simulink model "S32K39_FaultLogic_NXP_Codegen"  (R2024a)
settings: Solver=FixedStepAuto  StartTime=0.0  StopTime=10.0  FixedStep=1  RelTol=1e-3
PreLoadFcn:
  | % NXP_MBDT_S32K3 callback: DO NOT REMOVE
  | mbd_s32k3.common.nxp.model_callbacks.preLoadFcn();
PostLoadFcn:
  | % NXP_MBDT_S32K3 callback: DO NOT REMOVE
  | mbd_s32k3.common.nxp.model_callbacks.postLoadFcn();
InitFcn:
  | % NXP_MBDT_S32K3 callback: DO NOT REMOVE
  | mbd_s32k3.common.nxp.model_callbacks.initFcn();
settings Model: DataDictionary=S32K39_FaultLogic_NXP_Codegen.sldd  Creator=nxf64875  LastModifiedBy=nxf64875
settings DataIOCC: SaveOutput=off  SaveTime=off
settings OptimizationCC: EnhancedBackFolding=on  PassReuseOutputArgsAs=Individual arguments  ZeroExternalMemoryAtStartup=off  ZeroInternalMemoryAtStartup=off  MaxStackSize=64  OptimizeBlockOrder=speed  DifferentSizesBufferReuse=on  OptimizationCustomize=off  EfficientTunableParamExpr=on
settings DebuggingCC: ParameterTunabilityLossMsg=error
settings HardwareCC: ProdBitPerPointer=32  ProdBitPerSizeT=32  ProdBitPerPtrDiffT=32  ProdLargestAtomicInteger=Long  ProdLargestAtomicFloat=Double  ProdWordSize=32  ProdHWDeviceType=ARM Compatible->ARM Cortex
settings SFSimCC: MATLABDynamicMemAlloc=off
settings RTWCC: Description=Embedded Coder  SystemTargetFile=ert.tlc  HardwareBoard=NXP S32K3xx  TemplateMakefile=ert_default_tmf  Toolchain=S32DS GCC  BuildConfiguration=Faster Runs  CodeExecutionProfiling=on  CodeProfilingInstrumentation=coarse
settings CodeAppCC: ForceParamTrailComments=on  IgnoreCustomStorageClasses=off  OperatorAnnotations=on  SimulinkDataObjDesc=on  SFDataObjDesc=on  InsertBlockDesc=on
settings ERTTargetCC: ExtModeTransport=1  ExtModeMexFile=ext_serial_win32_comm  ERTSrcFileBannerTemplate=mbd_s32k3_ert_code_template.cgt  ERTHdrFileBannerTemplate=mbd_s32k3_ert_code_template.cgt  ERTDataSrcFileTemplate=mbd_s32k3_ert_code_template.cgt  ERTDataHdrFileTemplate=mbd_s32k3_ert_code_template.cgt

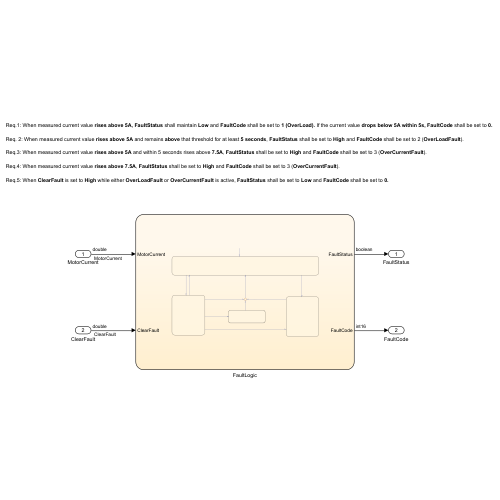
[thumbnail: Simulink's stored preview of the top-level diagram]
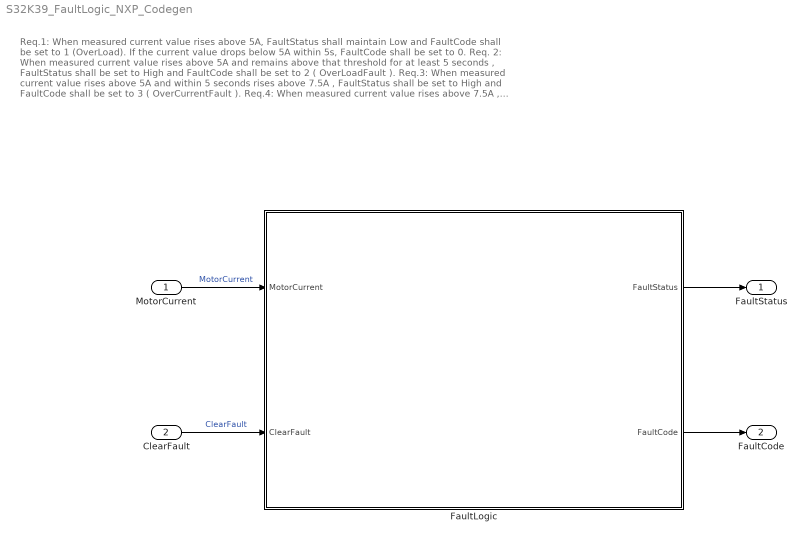
== system S32K39_FaultLogic_NXP_Codegen ==
  note: Req.1: When measured current value rises above 5A, FaultStatus shall maintain Low and FaultCode shall be set to 1 (OverLoad). If the current value drops below 5A within 5s, FaultCode shall be set to 0.
      |
      | Req. 2: When measured current value rises above 5A and remains above that threshold for at least 5 seconds , FaultStatus shall be set to High and FaultCode shall be set to 2 ( OverLoadFault ).
      |
      | Req.3: When measured current value rises above 5A and within 5 seconds rises above 7.5A , FaultStatus shall be set to High and FaultCode shall be set to 3 ( OverCurrentFault ).
      |
      | Req.4: When measured current value rises above 7.5A , FaultStatus shall be set to High and FaultCode shall be set to 3 ( OverCurrentFault ).
      |
      | Req.5: When ClearFault is set to High while either OverLoadFault or OverCurrentFault is active, FaultStatus shall be set to Low and FaultCode shall be set to 0.
  MotorCurrent : Inport
  ClearFault : Inport  Port=2
  FaultLogic : Stateflow chart  TreatAsAtomicUnit=on
  FaultStatus : Outport
  FaultCode : Outport  Port=2
  wires:
  MotorCurrent/1 -> FaultLogic/1(MotorCurrent)  "MotorCurrent"
  ClearFault/1 -> FaultLogic/2(ClearFault)  "ClearFault"
  FaultLogic/1(FaultStatus) -> FaultStatus/1
  FaultLogic/2(FaultCode) -> FaultCode/1

== stateflow chart S32K39_FaultLogic_NXP_Codegen/FaultLogic ==
  state NoFault
    entry:
    FaultCode = int16(0);
    FaultStatus = false;
  state OverLoad
    entry:
    FaultCode = int16(1);
    FaultStatus = false;
  state OverCurrentFault
    entry:
    FaultCode = int16(3);
    FaultStatus = true;
  state OverLoadFault
    entry:
    FaultCode = int16(2);
    FaultStatus = true;
  (default) -> NoFault : %Entry
  NoFault -> OverLoad [order 2] : [MotorCurrent>=single(5)]
  OverLoad -> NoFault [order 3] : [MotorCurrent<single(5)]
  (junction 35) -> NoFault
  NoFault -> OverCurrentFault [order 1] : [MotorCurrent > single(7.5)]
  OverLoad -> (junction 35) [order 1] : [ClearFault]
  OverCurrentFault -> (junction 35) : [ClearFault]
  OverLoadFault -> (junction 35) : [ClearFault]
  OverLoad -> OverLoadFault [order 4] : [elapsed(sec) > 5]
  OverLoad -> OverCurrentFault [order 2] : [MotorCurrent > single(7.5)]
  data: FaultStatus output boolean; FaultCode output int16; MotorCurrent input single; ClearFault input boolean
